simulink model "solution"  (R2018b)
settings: Solver=VariableStepAuto  StartTime=0.0  StopTime=Tmax-0.01  FixedStep=0.01  RelTol=1e-3
undefined symbols (not defined in the file): a0val, a_opt_fun, afval, j_opt_fun, s_opt_fun, Tmax, v0val, v_opt_fun, vfval, xfval
settings Model: Creator=tonegas  LastModifiedBy=tonegas

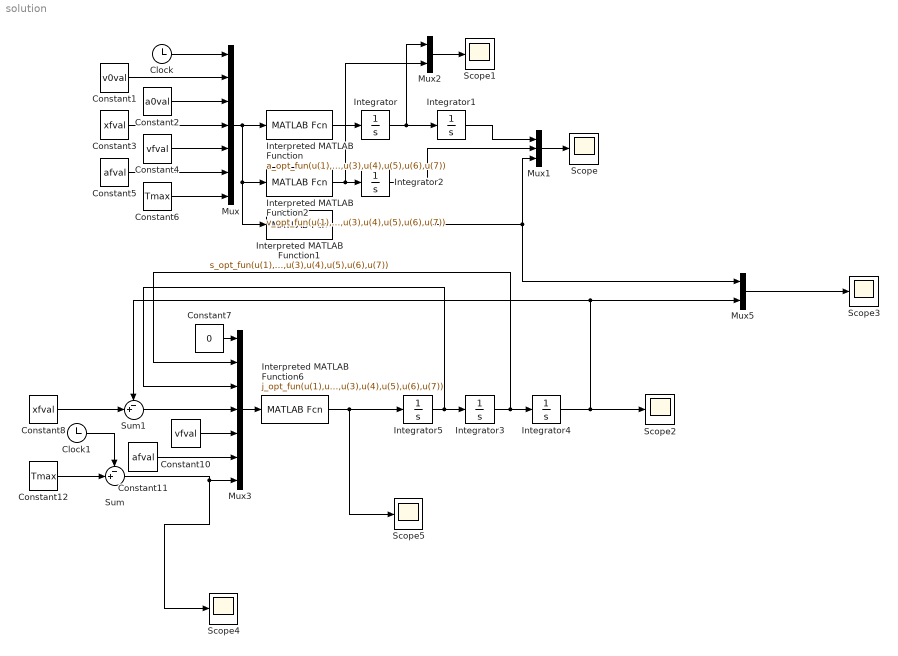
== system solution ==
  Clock : Clock
  Clock1 : Clock
  Constant1 : Constant  Value=v0val
  Constant10 : Constant  Value=vfval
  Constant11 : Constant  Value=afval
  Constant12 : Constant  Value=Tmax
  Constant2 : Constant  Value=a0val
  Constant3 : Constant  Value=xfval
  Constant4 : Constant  Value=vfval
  Constant5 : Constant  Value=afval
  Constant6 : Constant  Value=Tmax
  Constant7 : Constant  Value=0
  Constant8 : Constant  Value=xfval
  Integrator : Integrator  InitialCondition=v0val
  Integrator1 : Integrator
  Integrator2 : Integrator
  Integrator3 : Integrator  InitialCondition=v0val
  Integrator4 : Integrator
  Integrator5 : Integrator  InitialCondition=a0val
  Interpreted MATLAB Function : MATLABFcn  MATLABFcn=a_opt_fun(u(1),u(2),u(3),u(4),u(5),u(6),u(7))  OutputDimensions=1
  Interpreted MATLAB Function1 : MATLABFcn  MATLABFcn=s_opt_fun(u(1),u(2),u(3),u(4),u(5),u(6),u(7))  OutputDimensions=1
  Interpreted MATLAB Function2 : MATLABFcn  MATLABFcn=v_opt_fun(u(1),u(2),u(3),u(4),u(5),u(6),u(7))  OutputDimensions=1
  Interpreted MATLAB Function6 : MATLABFcn  MATLABFcn=j_opt_fun(u(1),u(2),u(3),u(4),u(5),u(6),u(7))  OutputDimensions=1
  Mux : Mux  Inputs=7
  Mux1 : Mux  Inputs=3
  Mux2 : Mux  Inputs=2
  Mux3 : Mux  Inputs=7
  Mux5 : Mux  Inputs=2
  Scope{,1..5} (6 alike) : Scope
  Sum : Sum  Inputs=-+|
  Sum1 : Sum  Inputs=-+|
  wires:
  Mux/1 -> Interpreted MATLAB Function2/1, Interpreted MATLAB Function1/1, Interpreted MATLAB Function/1
  Clock/1 -> Mux/1
  Constant1/1 -> Mux/2
  Constant2/1 -> Mux/3
  Constant3/1 -> Mux/4
  Constant4/1 -> Mux/5
  Constant5/1 -> Mux/6
  Constant6/1 -> Mux/7
  Integrator/1 -> Mux2/1, Integrator1/1
  Interpreted MATLAB Function1/1 -> Mux5/1, Mux1/3
  Mux1/1 -> Scope/1
  Interpreted MATLAB Function/1 -> Integrator/1
  Interpreted MATLAB Function2/1 -> Mux2/2, Integrator2/1
  Integrator2/1 -> Mux1/2
  Integrator1/1 -> Mux1/1
  Mux2/1 -> Scope1/1
  Constant11/1 -> Mux3/6
  Clock1/1 -> Sum/1
  Sum1/1 -> Mux3/4
  Sum/1 -> Scope4/1, Mux3/7
  Constant10/1 -> Mux3/5
  Mux5/1 -> Scope3/1
  Constant7/1 -> Mux3/1
  Mux3/1 -> Interpreted MATLAB Function6/1
  Constant12/1 -> Sum/2
  Constant8/1 -> Sum1/2
  Integrator3/1 -> Integrator4/1, Mux3/2
  Integrator5/1 -> Mux3/3, Integrator3/1
  Integrator4/1 -> Mux5/2, Sum1/1, Scope2/1
  Interpreted MATLAB Function6/1 -> Integrator5/1, Scope5/1
